simulink model "Learning_project_1"  (R2021a)
settings: Solver=VariableStepAuto  StartTime=0.0  StopTime=10.0  MaxStep=0.01  RelTol=1e-3
settings Model: Creator=tanmoyera  LastModifiedBy=tanmoyera

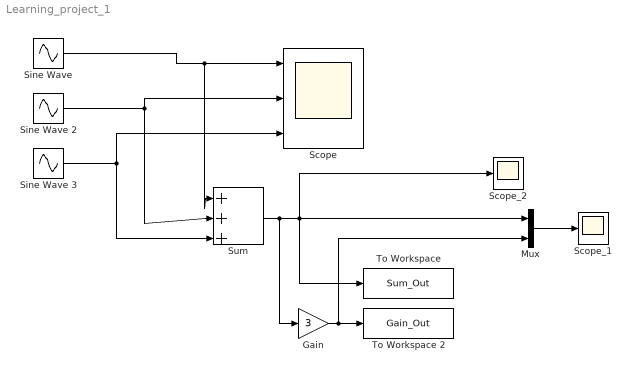
== system Learning_project_1 ==
  Gain : Gain  Gain=3
  Mux : Mux  Inputs=2
  "Scope " : Scope  NumInputPorts=3
  Scope_1 : Scope
  Scope_2 : Scope
  "Sine Wave " : Sin  SampleTime=0
  Sine Wave 2 : Sin  Frequency=5  SampleTime=0
  Sine Wave 3 : Sin  Frequency=10  SampleTime=0
  Sum : Sum  Inputs=|+++
  To Workspace : ToWorkspace  VariableName=Sum_Out  SaveFormat=Timeseries  SampleTime=-1
  To Workspace 2 : ToWorkspace  VariableName=Gain_Out  SaveFormat=Timeseries  SampleTime=-1
  wires:
  "Sine Wave "/1 -> Sum/1, "Scope "/1
  Sine Wave 2/1 -> Sum/2, "Scope "/2
  Sine Wave 3/1 -> Sum/3, "Scope "/3
  Sum/1 -> Gain/1, To Workspace/1, Mux/1, Scope_2/1
  Gain/1 -> Mux/2, To Workspace 2/1
  Mux/1 -> Scope_1/1
